simulink model "CompensationLoopModel"  (R2017b)
settings: Solver=VariableStepAuto  StartTime=0.0  StopTime=10  RelTol=1e-3
values from neighbouring files (symbols this model uses):
  s = tf('s')    [BoostModel.m]    (also in BoostModelSipex.m; BoostModelStandard.m)
libraries: slctrlblks x1
settings Model: Creator=Matt  LastModifiedBy=Matt

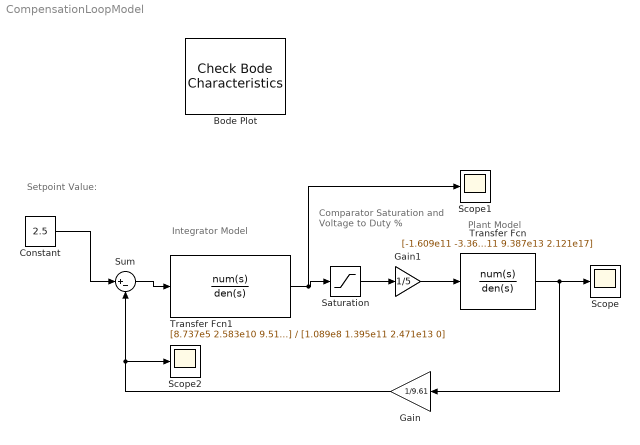
== system CompensationLoopModel ==
  note: Plant Model
  note: Comparator Saturation
      | and Voltage to Duty %
  note: Integrator Model
  note: Setpoint Value:
  Bode Plot : slctrlblks/Model Verification/Check Bode  Characteristics  InstantiateOnLoad=on  SaveOperatingPoints=off  LinearizationIOs={'/Transfer Fcn', 1, 'out', 'off', '';'/Constant', 1, 'in', 'off', ''}  LinearizeAt=SnapshotTimes  SnapshotTimes=[0]  TriggerType=rising  SampleTime=auto  RateConversionMethod=zoh  PreWarpFreq=10  UseExactDelayModel=off  UseFullBlockNameLabels=off  UseBusSignalLabels=off  enabled=on  stopWhenAssertionFail=off  export=off  ViewDlgPos=[100 106 555.5 484]  OpenViewOnLoad=off  LaunchViewOnOpen=off  FrequencyUnits=rad/s  MagnitudeUnits=dB  PhaseUnits=deg  TimeUnits=seconds  EnableUpperBound=off  UpperBoundFrequencies=[]  UpperBoundMagnitudes=[]  EnableLowerBound=off  LowerBoundFrequencies=[]  LowerBoundMagnitudes=[]
      settings: SourceProductName=Simulink Control Design
  Constant : Constant  Value=2.5
  Gain : Gain  Gain=1/9.61
  Gain1 : Gain  Gain=1/5
  Saturation : Saturate  UpperLimit=5  LowerLimit=0
  Scope : Scope
  Scope1 : Scope
  Scope2 : Scope
  Sum : Sum  Inputs=|+-
  Transfer Fcn : TransferFcn  Numerator=[-1.609e11 -3.369e15 1.753e19]  Denominator=[2.462e11 9.387e13 2.121e17]
  Transfer Fcn1 : TransferFcn  Numerator=[8.737e5 2.583e10 9.519e13]  Denominator=[1.089e8 1.395e11 2.471e13 0]
  wires:
  Constant/1 -> Sum/1
  Transfer Fcn/1 -> Scope/1, Gain/1
  Saturation/1 -> Gain1/1
  Gain1/1 -> Transfer Fcn/1
  Gain/1 -> Scope2/1, Sum/2
  Sum/1 -> Transfer Fcn1/1
  Transfer Fcn1/1 -> Scope1/1, Saturation/1
